simulink model "F28379DFirmware"  (R2023b)
settings: Solver=FixedStepAuto  StartTime=0.0  StopTime=Inf  FixedStep=5e-5  RelTol=1e-3  EnableMultiTasking=on
undefined symbols (not defined in the file): DiscIntNeverNeededParam, Down, F28379D_ADC_MaxCount, F28379D_ADC_Vmax, F28379D_PWM_Counter_Period, Foc_Ki_IxTcpu, Foc_Ki_S, Foc_Kp_I, Foc_Kp_S, GPTRIP1SEL, GPTRIP2SEL, Ia_offset, Ib_offset, IO334_DAC_Vmax, Maxon_645604_Np, PU_System_I_base, PU_System_N_base, Ts_CPU, TZ1, TZ2, Up
libraries: mcbcontrolslib x11, c280xlib x8, canmsglib x7, c2802xlib x6, slpidlib x3, simulink x3, mcbpositiondecoderlib x3, c2837xDlib x3
(part 1 of 2)
settings Model: DataDictionary=PMSM3P2LInverterDd.sldd  EnableAccessToBaseWorkspace=off  ExtModeTrigDuration=8  Creator=mathieu.lu-dac  LastModifiedBy=mathieu.lu-dac
settings OptimizationCC: DefaultUnderspecifiedDataType=single  EnhancedBackFolding=on  PassReuseOutputArgsAs=Individual arguments  MaxStackSize=1024  OptimizeBlockOrder=speed  DifferentSizesBufferReuse=on  OptimizationCustomize=off  DenormalBehavior=FlushToZero  EfficientTunableParamExpr=on
settings DebuggingCC: ParameterTunabilityLossMsg=error
settings HardwareCC: ProdBitPerChar=16  ProdBitPerInt=16  ProdBitPerPointer=32  ProdBitPerSizeT=32  ProdBitPerPtrDiffT=32  ProdLargestAtomicInteger=Integer  ProdLargestAtomicFloat=None  ProdWordSize=16  ProdLongLongMode=on  ProdHWDeviceType=Texas Instruments->C2000
settings SFSimCC: MATLABDynamicMemAlloc=off
settings RTWCC: Description=Embedded Coder  SystemTargetFile=ert.tlc  HardwareBoard=TI Delfino F28379D LaunchPad  TemplateMakefile=ert_default_tmf  Toolchain=Texas Instruments Code Composer Studio (C2000)  PortableWordSizes=on
settings CodeAppCC: ForceParamTrailComments=on  IgnoreCustomStorageClasses=off  OperatorAnnotations=on  SimulinkDataObjDesc=on  SFDataObjDesc=on  InsertBlockDesc=on
settings ERTTargetCC: CodeReplacementLibrary=TI C28x  SupportContinuousTime=on  ExtModeTransport=4  ExtModeStaticAlloc=on  ExtModeAutomaticAllocSize=off  ExtModeMexFile=ext_xcp  ExtModeIntrfLevel=Level2 - Open

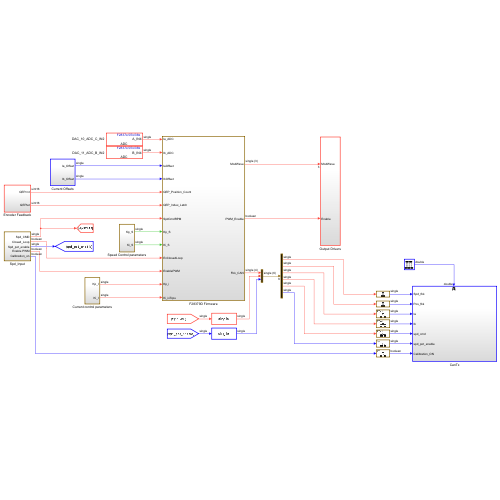
[thumbnail: Simulink's stored preview of the top-level diagram]
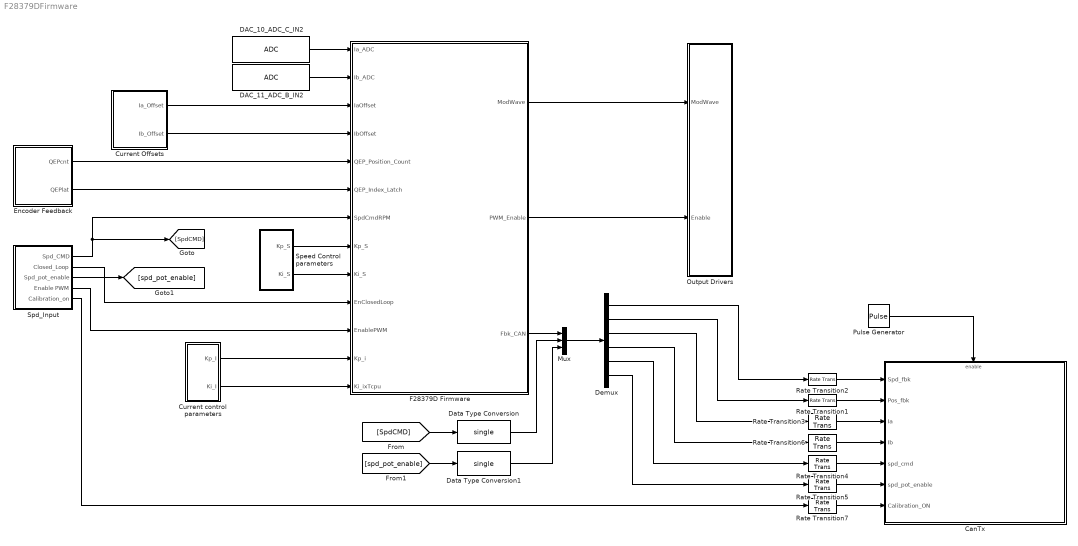
== system F28379DFirmware ==
  CanTx : Subsystem
  Current Offsets : Subsystem
  Current control parameters : Subsystem
  DAC_10_ADC_C_IN2 : c2802xlib/ADC  blkParamProc=C2000_Type4  ADCModule=A  samplingMode=Single sample mode  ADCResolution=12-bit (Single-ended input)  useSOC1=SOC0  useSOC2=SOC0_SOC1  SOCAcquisitionWindow=15  SOCTriggerSource=ePWM1_ADCSOCA  SOCInterruptTrigger=No ADCINT  Ts=-1  dType=single  postInterrupt=off  interruptSel=ADCINT1  ADCINTContinuous=on  endma=off  chdma=1  conv1=ADCINA0  conv2=ADCINA0 and ADCINB0  conv1_Type4=ADCIN4  conv2_Type4=ADCIN0 and ADCIN1
  DAC_11_ADC_B_IN2 : c2802xlib/ADC  blkParamProc=C2000_Type4  ADCModule=B  samplingMode=Single sample mode  ADCResolution=12-bit (Single-ended input)  useSOC1=SOC0  useSOC2=SOC0_SOC1  SOCAcquisitionWindow=15  SOCTriggerSource=ePWM1_ADCSOCA  SOCInterruptTrigger=No ADCINT  Ts=-1  dType=single  postInterrupt=on  interruptSel=ADCINT1  ADCINTContinuous=on  endma=off  chdma=1  conv1=ADCINA0  conv2=ADCINA0 and ADCINB0  conv1_Type4=ADCIN4  conv2_Type4=ADCIN0 and ADCIN1
  Data Type Conversion : DataTypeConversion  OutDataTypeStr=single  SaturateOnIntegerOverflow=off  RndMeth=Floor
  Data Type Conversion1 : DataTypeConversion  OutDataTypeStr=single  SaturateOnIntegerOverflow=off  RndMeth=Floor
  Demux : Demux  Outputs=6
  Encoder Feedback : Subsystem
  F28379D Firmware : Subsystem
  Mux : Mux  Inputs=3
  Output Drivers : Subsystem
  Pulse Generator : DiscretePulseGenerator  Period=10  PulseWidth=5  SampleTime=-1
  Rate Transition{1..7} (7 alike) : RateTransition  OutPortSampleTime=1e-3
  Spd_Input : Subsystem
  Speed Control parameters : Subsystem
  wires:
  Pulse Generator/1 -> CanTx/Enable
  Rate Transition2/1 -> CanTx/1(Spd_fbk)
  Rate Transition1/1 -> CanTx/2(Pos_fbk)
  F28379D Firmware/2(PWM_Enable) -> Output Drivers/2(Enable)
  F28379D Firmware/1(ModWave) -> Output Drivers/1(ModWave)
  Rate Transition3/1 -> CanTx/3(Ia)
  DAC_11_ADC_B_IN2/1 -> F28379D Firmware/2(Ib_ADC)
  DAC_10_ADC_C_IN2/1 -> F28379D Firmware/1(Ia_ADC)
  Spd_Input/1(Spd_CMD) -> F28379D Firmware/7(SpdCmdRPM), [SpdCMD]
  Speed Control parameters/1(Kp_S) -> F28379D Firmware/8(Kp_S)
  Speed Control parameters/2(Ki_S) -> F28379D Firmware/9(Ki_S)
  Spd_Input/2(Closed_Loop) -> F28379D Firmware/10(EnClosedLoop)
  Spd_Input/4(Enable PWM) -> F28379D Firmware/11(EnablePWM)
  Rate Transition4/1 -> CanTx/5(spd_cmd)
  Rate Transition5/1 -> CanTx/6(spd_pot_enable)
  Demux/1 -> Rate Transition2/1
  Demux/2 -> Rate Transition1/1
  Rate Transition6/1 -> CanTx/4("Ib ")
  Demux/5 -> Rate Transition4/1
  Demux/6 -> Rate Transition5/1
  Current Offsets/1(Ia_Offset) -> F28379D Firmware/3(IaOffset)
  Current Offsets/2(Ib_Offset) -> F28379D Firmware/4(IbOffset)
  Demux/3 -> Rate Transition3/1
  Demux/4 -> Rate Transition6/1
  Current control parameters/1(Kp_I) -> F28379D Firmware/12(Kp_i)
  Current control parameters/2(Ki_I) -> F28379D Firmware/13(Ki_ixTcpu)
  Encoder Feedback/1(QEPcnt) -> F28379D Firmware/5(QEP_Position_Count)
  Encoder Feedback/2(QEPlat) -> F28379D Firmware/6(QEP_Index_Latch)
  F28379D Firmware/3(Fbk_CAN) -> Mux/1
  Mux/1 -> Demux/1
  Spd_Input/3(Spd_pot_enable) -> [spd_pot_enable]
  [SpdCMD] -> Data Type Conversion/1
  [spd_pot_enable] -> Data Type Conversion1/1
  Data Type Conversion/1 -> Mux/2
  Data Type Conversion1/1 -> Mux/3
  Spd_Input/5(Calibration_on) -> Rate Transition7/1
  Rate Transition7/1 -> CanTx/7(Calibration_ON)

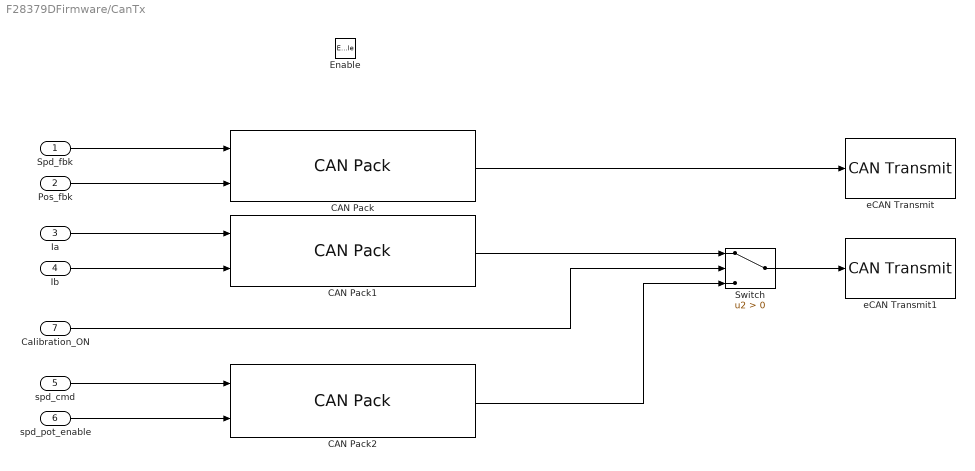
== system F28379DFirmware/CanTx ==
  Spd_fbk : Inport
  Pos_fbk : Inport  Port=2
  Ia : Inport  Port=3
  "Ib " : Inport  Port=4
  spd_cmd : Inport  Port=5
  spd_pot_enable : Inport  Port=6
  Calibration_ON : Inport  Port=7
  Enable : EnablePort
  CAN Pack : canmsglib/CAN Pack  MsgList=(none)  MsgName=Speed_TI_Out  MsgIDType=Standard (11-bit identifier)  MsgIdentifier=1  MsgLength=8  Remote=off  ApplyMinMax=off  BusOutput=off  SignalInfo={ 'Speed_fbk', '0', '32', 'LE', 'single', 'Standard', '0', '1', '0', '-Inf', 'Inf'; 'Pos_fbk', '32', '32', 'LE', 'single', 'Standard', '0', '1', '0', '-Inf', 'Inf' }
      settings: LibrarySourceBlock=canlib/CAN Pack  DataFormat=manually specified signals
  CAN Pack1 : canmsglib/CAN Pack  MsgList=(none)  MsgName=I_TI_Out  MsgIDType=Standard (11-bit identifier)  MsgIdentifier=2  MsgLength=8  Remote=off  ApplyMinMax=off  BusOutput=off  SignalInfo={ 'Ia', '0', '32', 'LE', 'single', 'Standard', '0', '1', '0', '-Inf', 'Inf'; 'Ib', '32', '32', 'LE', 'single', 'Standard', '0', '1', '0', '-Inf', 'Inf' }
      settings: LibrarySourceBlock=canlib/CAN Pack  DataFormat=manually specified signals
  CAN Pack2 : canmsglib/CAN Pack  MsgList=(none)  MsgName=Debug_TI_Out  MsgIDType=Standard (11-bit identifier)  MsgIdentifier=2  MsgLength=8  Remote=off  ApplyMinMax=off  BusOutput=off  SignalInfo={ 'spd_cmd', '0', '32', 'LE', 'single', 'Standard', '0', '1', '0', '-Inf', 'Inf'; 'spd_pot_enable', '32', '32', 'LE', 'single', 'Standard', '0', '1', '0', '-Inf', 'Inf' }
      settings: LibrarySourceBlock=canlib/CAN Pack  DataFormat=manually specified signals
  Switch : Switch  Criteria=u2 > Threshold  SaturateOnIntegerOverflow=off  InputSameDT=off
  eCAN Transmit : c280xlib/CAN Transmit  chipFamily=C280x  useModule=CAN_B  mailboxNo=1  messageID=1  messageType=Standard (11-bit identifier)  enableBlockingMode=off  postInterrupt=off  interruptLine=0
  eCAN Transmit1 : c280xlib/CAN Transmit  chipFamily=C280x  useModule=CAN_B  mailboxNo=1  messageID=2  messageType=Standard (11-bit identifier)  enableBlockingMode=off  postInterrupt=off  interruptLine=0
  wires:
  CAN Pack/1 -> eCAN Transmit/1
  Spd_fbk/1 -> CAN Pack/1
  Pos_fbk/1 -> CAN Pack/2
  Ia/1 -> CAN Pack1/1
  "Ib "/1 -> CAN Pack1/2
  spd_cmd/1 -> CAN Pack2/1
  spd_pot_enable/1 -> CAN Pack2/2
  Switch/1 -> eCAN Transmit1/1
  Calibration_ON/1 -> Switch/2
  CAN Pack1/1 -> Switch/1
  CAN Pack2/1 -> Switch/3

== system F28379DFirmware/Current Offsets ==
  CAN Unpack1 : canmsglib/CAN Unpack  MsgList=(none)  MsgName=CAN Msg  MsgIDType=Standard (11-bit identifier)  MsgIdentifier=30  MsgLength=8  SignalInfo={ 'Ia_off', '0', '32', 'LE', 'single', 'Standard', '0', '1', '0', '-Inf', 'Inf'; 'Ib_off', '32', '32', 'LE', 'single', 'Standard', '0', '1', '0', '-Inf', 'Inf' }  IDPort=off  TimestampPort=off  ErrorPort=off  RemotePort=off  LengthPort=off  StatusPort=off  ApplyMinMax=off
      settings: LibrarySourceBlock=canlib/CAN Unpack
  Data Type Conversion : DataTypeConversion  OutDataTypeStr=single  SaturateOnIntegerOverflow=off  RndMeth=Floor
  Data Type Conversion1 : DataTypeConversion  OutDataTypeStr=single  SaturateOnIntegerOverflow=off  RndMeth=Floor
  Ia Offset : Constant  Value=Ia_offset
  Ib Offset : Constant  Value=Ib_offset
  Switch : Switch  Criteria=u2 ~= 0  SaturateOnIntegerOverflow=off  InputSameDT=off
  Switch1 : Switch  Criteria=u2 ~= 0  SaturateOnIntegerOverflow=off  InputSameDT=off
  eCAN Receive ADC_OFFsets1 : c280xlib/CAN Receive  chipFamily=C280x  useModule=CAN_B  mailboxNo=30  messageID=30  messageType=Standard (11-bit identifier)  enableAcceptanceFiltering=off  messageIDMask=0  sampleTime=0.1  dataType=CAN_MESSAGE_TYPE  outputAction=Output last received values  initValue=0  outputMessageID=off  outputMessageLength=off  outputMessageTimeStamp=off  postInterrupt=off  interruptLine=0
  Ia_Offset : Outport
  Ib_Offset : Outport  Port=2
  wires:
  eCAN Receive ADC_OFFsets1/2 -> CAN Unpack1/1
  Switch/1 -> Data Type Conversion/1
  Switch1/1 -> Data Type Conversion1/1
  Ia Offset/1 -> Switch/3
  Ib Offset/1 -> Switch1/3
  CAN Unpack1/1 -> Switch/2, Switch/1
  CAN Unpack1/2 -> Switch1/1, Switch1/2
  Data Type Conversion/1 -> Ia_Offset/1
  Data Type Conversion1/1 -> Ib_Offset/1

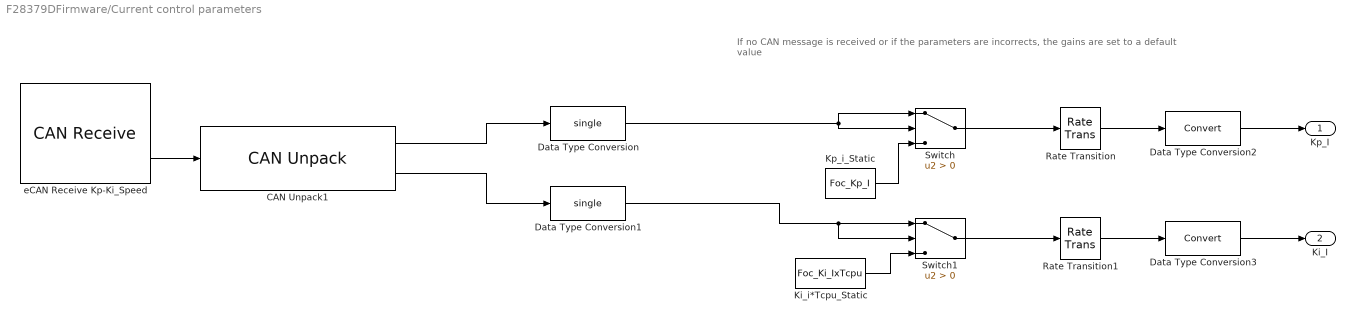
== system F28379DFirmware/Current control parameters ==
  note: If no CAN message is received or if the parameters are incorrects, the gains are set to a default value
  CAN Unpack1 : canmsglib/CAN Unpack  MsgList=(none)  MsgName=CAN Msg  MsgIDType=Standard (11-bit identifier)  MsgIdentifier=29  MsgLength=8  SignalInfo={ 'Kp_I', '0', '32', 'LE', 'single', 'Standard', '0', '1', '0', '-Inf', 'Inf'; 'Ki_I', '32', '32', 'LE', 'single', 'Standard', '0', '1', '0', '-Inf', 'Inf' }  IDPort=off  TimestampPort=off  ErrorPort=off  RemotePort=off  LengthPort=off  StatusPort=off  ApplyMinMax=off
      settings: LibrarySourceBlock=canlib/CAN Unpack
  Data Type Conversion : DataTypeConversion  OutDataTypeStr=single  SaturateOnIntegerOverflow=off  RndMeth=Floor
  Data Type Conversion1 : DataTypeConversion  OutDataTypeStr=single  SaturateOnIntegerOverflow=off  RndMeth=Floor
  Data Type Conversion2 : DataTypeConversion  SaturateOnIntegerOverflow=off  RndMeth=Floor
  Data Type Conversion3 : DataTypeConversion  SaturateOnIntegerOverflow=off  RndMeth=Floor
  Ki_i*Tcpu_Static : Constant  Value=Foc_Ki_IxTcpu  OutDataTypeStr=single  SampleTime=-1
  Kp_i_Static : Constant  Value=Foc_Kp_I  OutDataTypeStr=single  SampleTime=-1
  Rate Transition : RateTransition
  Rate Transition1 : RateTransition  InitialCondition=Ts_CPU
  Switch : Switch  Criteria=u2 > Threshold  SaturateOnIntegerOverflow=off  InputSameDT=off
  Switch1 : Switch  Criteria=u2 > Threshold  SaturateOnIntegerOverflow=off  InputSameDT=off
  eCAN Receive Kp-Ki_Speed : c280xlib/CAN Receive  chipFamily=C280x  useModule=CAN_B  mailboxNo=29  messageID=29  messageType=Standard (11-bit identifier)  enableAcceptanceFiltering=off  messageIDMask=0  sampleTime=1e-3  dataType=CAN_MESSAGE_TYPE  outputAction=Output last received values  initValue=0  outputMessageID=off  outputMessageLength=off  outputMessageTimeStamp=off  postInterrupt=off  interruptLine=0
  Kp_I : Outport
  Ki_I : Outport  Port=2
  wires:
  Data Type Conversion3/1 -> Ki_I/1
  Data Type Conversion2/1 -> Kp_I/1
  Rate Transition1/1 -> Data Type Conversion3/1
  Rate Transition/1 -> Data Type Conversion2/1
  Ki_i*Tcpu_Static/1 -> Switch1/3
  Kp_i_Static/1 -> Switch/3
  Switch1/1 -> Rate Transition1/1
  Switch/1 -> Rate Transition/1
  Data Type Conversion1/1 -> Switch1/1, Switch1/2
  Data Type Conversion/1 -> Switch/2, Switch/1
  CAN Unpack1/2 -> Data Type Conversion1/1
  CAN Unpack1/1 -> Data Type Conversion/1
  eCAN Receive Kp-Ki_Speed/2 -> CAN Unpack1/1

== system F28379DFirmware/Encoder Feedback ==
  Data Type Conversion : DataTypeConversion  OutDataTypeStr=uint16  SaturateOnIntegerOverflow=off  RndMeth=Floor
  Data Type Conversion1 : DataTypeConversion  OutDataTypeStr=uint16  SaturateOnIntegerOverflow=off  RndMeth=Floor
  eQEP : c280xlib/eQEP  useModule=eQEP1  pcInputmode=Quadrature-count  externalClockrate=2x resolution: Count the rising/falling edge  swapPolarityselection=Clockwise  qdfOutputport=off  qapPolarityselection=off  qbpPolarityselection=off  qipPolarityselection=off  qspPolarityselection=off  igatePolarityselection=off  sampleTime=-1  pcOutputport=on  pcMaximumvalue=2^16-1  indexInitializationcheck=off  indexInitializationevent=Rising edge  strobeInitializationcheck=off  strobeInitializationevent=Rising edge  softwareInitializationcheck=off  softwareInitializationsource=Set to init value at start up  softwareInitializationmode=on  pcInitialvalue=2147483648  pcResetmode=Reset on the first index event  ieloutputport=on  indexEventlatch=Falling edge  seloutputport=off  strobeEventlatch=Rising edge  pcefOutputport=off  enableEqepcapture=off  qctmrOutputport=off  qcprdOutputport=off  captureTimerprescaler=128  upEventprescaler=128  overflowErrorflag=off  directionErrorflag=off  captureTimerposition=On position counter read  unitTimerperiod=100000000  captureTimerlatch=off  capturePeriodlatch=off  positionCounterlatch=off  soenPolarityselection=off  spselPolarityselection=Index pin is used for sync output  compareValuesource=Specify via dialog  shadowMode=Load on QPOSCNT=0  compareValue=4294967295  syncOutputwidth=1  polaritySyncoutput=Active high  watchdogEnable=off  watchdogTimer=65535  outport1Datatype=auto  outport2Datatype=auto  outport3Datatype=auto  outport4Datatype=auto  outport5Datatype=auto  outport6Datatype=auto  outport7Datatype=auto  outport8Datatype=auto  outport9Datatype=auto  outport10Datatype=auto  outport11Datatype=auto  outport12Datatype=auto  eqepinterrupt_pce=off  eqepinterrupt_qpe=off  eqepinterrupt_qdc=off  eqepinterrupt_wto=off  eqepinterrupt_pcu=off  eqepinterrupt_pco=off  eqepinterrupt_pcr=off  eqepinterrupt_pcm=off  eqepinterrupt_sel=off  eqepinterrupt_iel=off  eqepinterrupt_uto=off  pheOutputport=off  watchdogOutputport=off  outport13Datatype=auto  outport14Datatype=auto
  QEPcnt : Outport
  QEPlat : Outport  Port=2
  wires:
  eQEP/1 -> Data Type Conversion/1
  eQEP/2 -> Data Type Conversion1/1
  Data Type Conversion1/1 -> QEPlat/1
  Data Type Conversion/1 -> QEPcnt/1

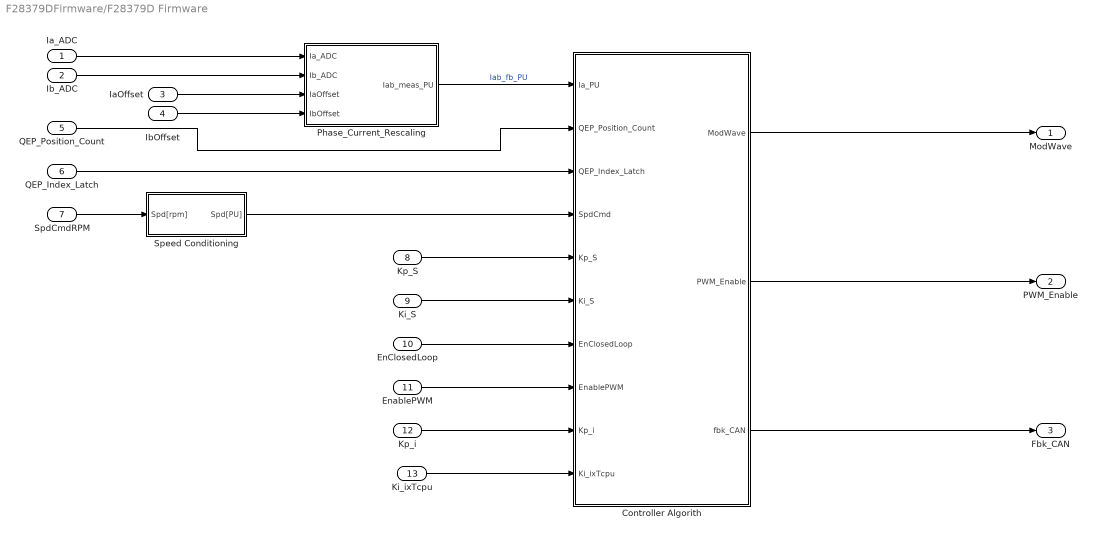
== system F28379DFirmware/F28379D Firmware ==
  Ia_ADC : Inport
  Ib_ADC : Inport  Port=2
  IaOffset : Inport  Port=3
  IbOffset : Inport  Port=4
  QEP_Position_Count : Inport  Port=5
  QEP_Index_Latch : Inport  Port=6
  SpdCmdRPM : Inport  Port=7
  Kp_S : Inport  Port=8
  Ki_S : Inport  Port=9
  EnClosedLoop : Inport  Port=10
  EnablePWM : Inport  Port=11
  Kp_i : Inport  Port=12
  Ki_ixTcpu : Inport  Port=13
  Controller Algorith : Subsystem
  Phase_Current_Rescaling : Subsystem
  Speed Conditioning : Subsystem
  ModWave : Outport
  PWM_Enable : Outport  Port=2
  Fbk_CAN : Outport  Port=3
  wires:
  SpdCmdRPM/1 -> Speed Conditioning/1(Spd[rpm])
  Ia_ADC/1 -> Phase_Current_Rescaling/1(Ia_ADC)
  IaOffset/1 -> Phase_Current_Rescaling/3(IaOffset)
  IbOffset/1 -> Phase_Current_Rescaling/4(IbOffset)
  QEP_Position_Count/1 -> Controller Algorith/2(QEP_Position_Count)
  Controller Algorith/1(ModWave) -> ModWave/1
  Phase_Current_Rescaling/1(Iab_meas_PU) -> Controller Algorith/1(Ia_PU)  "Iab_fb_PU"
  Kp_S/1 -> Controller Algorith/5(Kp_S)
  Controller Algorith/2(PWM_Enable) -> PWM_Enable/1
  Ki_S/1 -> Controller Algorith/6(Ki_S)
  QEP_Index_Latch/1 -> Controller Algorith/3(QEP_Index_Latch)
  Ib_ADC/1 -> Phase_Current_Rescaling/2(Ib_ADC)
  EnClosedLoop/1 -> Controller Algorith/7(EnClosedLoop)
  EnablePWM/1 -> Controller Algorith/8(EnablePWM)
  Speed Conditioning/1(Spd[PU]) -> Controller Algorith/4(SpdCmd)
  Controller Algorith/3(fbk_CAN) -> Fbk_CAN/1
  Kp_i/1 -> Controller Algorith/9(Kp_i)
  Ki_ixTcpu/1 -> Controller Algorith/10(Ki_ixTcpu)

== system F28379DFirmware/Output Drivers ==
  note: for inverter connected with LaunchXL-28379D
  note: System Outputs
  ModWave : Inport
  Enable : Inport  Port=2
  Demux1 : Demux  Outputs=3
  Mux3 : Mux  Inputs=3
  Scale_to_PWM_Counter_PRD : Gain  Gain=F28379D_PWM_Counter_Period  OutDataTypeStr=uint16  RndMeth=Simplest
  Switch1 : Switch  Threshold=0.5  SaturateOnIntegerOverflow=off  InputSameDT=off
  ePWM1 : c2802xlib/ePWM  PwmType=C2000_Type4  useModule=ePWM1  ePWMxLINKTBPRD=Not Linked  periodUnits=Clock cycles  timerSource=Specify via dialog  timerPeriod_clk=F28379D_PWM_Counter_Period+1  timerPeriod_sec=0.0001  tbshadow=Counter equals to zero  countingMode=Up-Down  phaseActiveEnable=Disable  phaseDirection=Count down after sync  phaseActive=0  synchronizationEnable=off  dcaevt1Sync=off  dcbevt1Sync=off  synchronizationOption=Counter equals to zero (CTR=Zero)  dcbevt1SyncOut=off  dcaevt1SyncOut=off  cmpdSyncOut=off  cmpcSyncOut=off  cmpbSyncOut=off  zeroSyncOut=on  swfSyncOut=off  perSynchronizationOption=Counter equals to period (CTR=PRD)  clockPrescale=1  HSclockPrescale=1  enswap=off  ePWMxAStatus=on  ePWMxAactionLogic1=Do nothing  ePWMxAactionLogic2=Do nothing  ePWMxAactionLogic3=Clear  ePWMxAactionLogic4=Set  ePWMxAactionLogic5=Do nothing  ePWMxAactionLogic6=Do nothing  ePWMxACSFenable=off  ePWMxACSFvalue=Forcing disable  ePWMxASFreload=Zero  ePWMxBStatus=on  ePWMxBactionLogic1=Set  ePWMxBactionLogic2=Clear  ePWMxBactionLogic3=Do nothing  ePWMxBactionLogic4=Do nothing  ePWMxBactionLogic5=Clear  ePWMxBactionLogic6=Set  ePWMxBCSFenable=off  ePWMxBCSFvalue=Forcing disable  ePWMxBSFreload=Zero  ePWNxBOutWay=on  ePWMxLINKCMPA=Not Linked  CMPAUnits=Clock cycles  CMPASource=Input port  CMPAValue_per=50  CMPAValue_clk=floor(F28379D_PWM_Counter_Period/2+1)  enCMPAshadow=Counter equals to zero (CTR=Zero)  ePWMxLINKCMPB=Not Linked  CMPBUnits=Clock cycles  CMPBSource=Specify via dialog  CMPBValue_per=50  CMPBValue_clk=floor(F28379D_PWM_Counter_Period/2+1)  enCMPBshadow=Counter equals to zero (CTR=Zero)  ePWMxLINKCMPC=Not Linked  CMPCUnits=Clock cycles  CMPCSource=Specify via dialog  CMPCValue_per=50  CMPCValue_clk=32000  enCMPCshadow=Counter equals to zero (CTR=Zero)  ePWMxLINKCMPD=Not Linked  CMPDUnits=Clock cycles  CMPDSource=Specify via dialog  CMPDValue_per=50  CMPDValue_clk=32000  enCMPDshadow=Counter equals to zero (CTR=Zero)  enableDBePWMxA=on  enableDBePWMxB=on  enhalfcycle=off  DBpolarity=Active high complementary (AHC)  DBedgeDelay=Positive  DBSource_ePWMxA=ePWMxA  DBSource_ePWMxB=ePWMxA  DBPeriodUnits=Clock cycles  DBperiodSource=Specify via dialog  REDperiod=15  FEDperiod=15  REDperiod_sec=0  FEDperiod_sec=0  LoadModeDBRED=Immediate without using shadow  LoadModeDBFED=Immediate without using shadow  adcstartModuleA=on  adcrequestEventA=First event  adcstartEventA=Digital Compare Module A Event 1 start of conversion (DCAEVT1.soc)  adcstartEventA_type2=Counter equals to period (CTR=PRD)  adcstartModuleB=off  adcrequestEventB=First event  adcstartEventB=Counter equals to zero (CTR=Zero)  adcstartEventB_type2=Counter equals to zero (CTR=Zero)  intEn=off  intPrd=First event  intSel=Counter equals to zero (CTR=Zero)  intSel_type2=Counter equals to zero (CTR=Zero)  hrpe=off  enHRPWM=off  HRPWM_LoadMode=Counter equals to period (CTR=PRD)  HRPWM_CTLMode=Duty or Period control mode  HRPWM_EDGMode=Both edge  hrpeb=off  enHRPWMB=off  HRPWM_LoadModeB=Counter equals to zero (CTR=ZERO)  HRPWM_CTLModeB=Duty or Period control mode  HRPWM_EDGModeB=Both edge  enHRDBRED=off  enHRDBFED=off  enSFO=on  enautoconv=on  chopperEnable=off  chopperFrequency=1  chopperFirstwidth=1  chopperDuty=12.5%  tripZonesource=Specify via dialog  tzselOSHT1=off  tzselOSHT2=off  tzselOSHT3=off  tzselOSHDCAEV1=off  tzselOSHDCBEV1=off  tzselCBC1=off  tzselCBC2=off  tzselCBC3=off  tzselCBCDCAEV2=off  tzselCBCDCBEV2=off  tzselOSHT4=off  tzselOSHT5=off  tzselOSHT6=off  tzselCBC4=off  tzselCBC5=off  tzselCBC6=off  enTzOstIntr=off  enTzCbcIntr=off  enTzDCAEVT1Intr=off  enTzDCAEVT2Intr=off  enTzDCBEVT1Intr=off  enTzDCBEVT2Intr=off  ePWMxAforced=No action  ePWMxBforced=No action  DCAEVT1forced=No action  DCBEVT1forced=No action  DCAEVT2forced=No action  DCBEVT2forced=No action  dcah=Trip Zone 1 input (TZ1)  dcal=Trip Zone 2 input (TZ2)  dcbh=Trip Zone 1 input (TZ1)  dcbl=Trip Zone 2 input (TZ2)  dcah_type2=GPTRIP1SEL/(TZ1)  dcal_type2=GPTRIP2SEL/(TZ2)  dcbh_type2=GPTRIP1SEL/(TZ1)  dcbl_type2=GPTRIP2SEL/(TZ2)  gendcaevt1=Event disabled  gendcaevt2=Event disabled  gendcbevt1=Event disabled  gendcbevt2=Event disabled  dcaevt1src=DCAEVT1 with sync  dcaevt2src=DCAEVT2 with sync  dcbevt1src=DCBEVT1 with sync  dcbevt2src=DCBEVT2 with sync  pulsesel=Counter equals to zero (CTR=Zero)  blankinv=off  blankoffset=0  blankwidth=0  evsrcsel=Filtered version of DCAEVT1 (DCAEVT1FILT)  encape=off
  ePWM2 : c2802xlib/ePWM  PwmType=C2000_Type4  useModule=ePWM2  ePWMxLINKTBPRD=Not Linked  periodUnits=Clock cycles  timerSource=Specify via dialog  timerPeriod_clk=F28379D_PWM_Counter_Period+1  timerPeriod_sec=0.0001  tbshadow=Counter equals to zero  countingMode=Up-Down  phaseActiveEnable=Set counter to phase value specified via dialog  phaseDirection=Count up after sync  phaseActive=0  synchronizationEnable=off  dcaevt1Sync=off  dcbevt1Sync=off  synchronizationOption=Pass through (EPWMxSYNCI or SWFSYNC)  dcbevt1SyncOut=off  dcaevt1SyncOut=off  cmpdSyncOut=off  cmpcSyncOut=off  cmpbSyncOut=off  zeroSyncOut=off  swfSyncOut=on  perSynchronizationOption=Counter equals to period (CTR=PRD)  clockPrescale=1  HSclockPrescale=1  enswap=off  ePWMxAStatus=on  ePWMxAactionLogic1=Do nothing  ePWMxAactionLogic2=Do nothing  ePWMxAactionLogic3=Clear  ePWMxAactionLogic4=Set  ePWMxAactionLogic5=Do nothing  ePWMxAactionLogic6=Do nothing  ePWMxACSFenable=off  ePWMxACSFvalue=Forcing disable  ePWMxASFreload=Zero  ePWMxBStatus=on  ePWMxBactionLogic1=Set  ePWMxBactionLogic2=Clear  ePWMxBactionLogic3=Do nothing  ePWMxBactionLogic4=Do nothing  ePWMxBactionLogic5=Clear  ePWMxBactionLogic6=Set  ePWMxBCSFenable=off  ePWMxBCSFvalue=Forcing disable  ePWMxBSFreload=Zero  ePWNxBOutWay=on  ePWMxLINKCMPA=Not Linked  CMPAUnits=Clock cycles  CMPASource=Input port  CMPAValue_per=50  CMPAValue_clk=floor(F28379D_PWM_Counter_Period/2+1)  enCMPAshadow=Counter equals to zero (CTR=Zero)  ePWMxLINKCMPB=Not Linked  CMPBUnits=Clock cycles  CMPBSource=Specify via dialog  CMPBValue_per=50  CMPBValue_clk=floor(F28379D_PWM_Counter_Period/2+1)  enCMPBshadow=Counter equals to zero (CTR=Zero)  ePWMxLINKCMPC=Not Linked  CMPCUnits=Clock cycles  CMPCSource=Specify via dialog  CMPCValue_per=50  CMPCValue_clk=32000  enCMPCshadow=Counter equals to zero (CTR=Zero)  ePWMxLINKCMPD=Not Linked  CMPDUnits=Clock cycles  CMPDSource=Specify via dialog  CMPDValue_per=50  CMPDValue_clk=32000  enCMPDshadow=Counter equals to zero (CTR=Zero)  enableDBePWMxA=on  enableDBePWMxB=on  enhalfcycle=off  DBpolarity=Active high complementary (AHC)  DBedgeDelay=Positive  DBSource_ePWMxA=ePWMxA  DBSource_ePWMxB=ePWMxA  DBPeriodUnits=Clock cycles  DBperiodSource=Specify via dialog  REDperiod=15  FEDperiod=15  REDperiod_sec=0  FEDperiod_sec=0  LoadModeDBRED=Immediate without using shadow  LoadModeDBFED=Immediate without using shadow  adcstartModuleA=off  adcrequestEventA=First event  adcstartEventA=Digital Compare Module A Event 1 start of conversion (DCAEVT1.soc)  adcstartEventA_type2=Counter equals to period (CTR=PRD)  adcstartModuleB=off  adcrequestEventB=First event  adcstartEventB=Counter equals to zero (CTR=Zero)  adcstartEventB_type2=Counter equals to zero (CTR=Zero)  intEn=off  intPrd=First event  intSel=Counter equals to zero (CTR=Zero)  intSel_type2=Counter equals to zero (CTR=Zero)  hrpe=off  enHRPWM=off  HRPWM_LoadMode=Counter equals to period (CTR=PRD)  HRPWM_CTLMode=Duty or Period control mode  HRPWM_EDGMode=Both edge  hrpeb=off  enHRPWMB=off  HRPWM_LoadModeB=Counter equals to zero (CTR=ZERO)  HRPWM_CTLModeB=Duty or Period control mode  HRPWM_EDGModeB=Both edge  enHRDBRED=off  enHRDBFED=off  enSFO=on  enautoconv=on  chopperEnable=off  chopperFrequency=1  chopperFirstwidth=1  chopperDuty=12.5%  tripZonesource=Specify via dialog  tzselOSHT1=off  tzselOSHT2=off  tzselOSHT3=off  tzselOSHDCAEV1=off  tzselOSHDCBEV1=off  tzselCBC1=off  tzselCBC2=off  tzselCBC3=off  tzselCBCDCAEV2=off  tzselCBCDCBEV2=off  tzselOSHT4=off  tzselOSHT5=off  tzselOSHT6=off  tzselCBC4=off  tzselCBC5=off  tzselCBC6=off  enTzOstIntr=off  enTzCbcIntr=off  enTzDCAEVT1Intr=off  enTzDCAEVT2Intr=off  enTzDCBEVT1Intr=off  enTzDCBEVT2Intr=off  ePWMxAforced=No action  ePWMxBforced=No action  DCAEVT1forced=No action  DCBEVT1forced=No action  DCAEVT2forced=No action  DCBEVT2forced=No action  dcah=Trip Zone 1 input (TZ1)  dcal=Trip Zone 2 input (TZ2)  dcbh=Trip Zone 1 input (TZ1)  dcbl=Trip Zone 2 input (TZ2)  dcah_type2=GPTRIP1SEL/(TZ1)  dcal_type2=GPTRIP2SEL/(TZ2)  dcbh_type2=GPTRIP1SEL/(TZ1)  dcbl_type2=GPTRIP2SEL/(TZ2)  gendcaevt1=Event disabled  gendcaevt2=Event disabled  gendcbevt1=Event disabled  gendcbevt2=Event disabled  dcaevt1src=DCAEVT1 with sync  dcaevt2src=DCAEVT2 with sync  dcbevt1src=DCBEVT1 with sync  dcbevt2src=DCBEVT2 with sync  pulsesel=Counter equals to zero (CTR=Zero)  blankinv=off  blankoffset=0  blankwidth=0  evsrcsel=Filtered version of DCAEVT1 (DCAEVT1FILT)  encape=off
  ePWM3 : c2802xlib/ePWM  PwmType=C2000_Type4  useModule=ePWM3  ePWMxLINKTBPRD=Not Linked  periodUnits=Clock cycles  timerSource=Specify via dialog  timerPeriod_clk=F28379D_PWM_Counter_Period+1  timerPeriod_sec=0.0001  tbshadow=Counter equals to zero  countingMode=Up-Down  phaseActiveEnable=Set counter to phase value specified via dialog  phaseDirection=Count up after sync  phaseActive=0  synchronizationEnable=off  dcaevt1Sync=off  dcbevt1Sync=off  synchronizationOption=Pass through (EPWMxSYNCI or SWFSYNC)  dcbevt1SyncOut=off  dcaevt1SyncOut=off  cmpdSyncOut=off  cmpcSyncOut=off  cmpbSyncOut=off  zeroSyncOut=off  swfSyncOut=on  perSynchronizationOption=Counter equals to period (CTR=PRD)  clockPrescale=1  HSclockPrescale=1  enswap=off  ePWMxAStatus=on  ePWMxAactionLogic1=Do nothing  ePWMxAactionLogic2=Do nothing  ePWMxAactionLogic3=Clear  ePWMxAactionLogic4=Set  ePWMxAactionLogic5=Do nothing  ePWMxAactionLogic6=Do nothing  ePWMxACSFenable=off  ePWMxACSFvalue=Forcing disable  ePWMxASFreload=Zero  ePWMxBStatus=on  ePWMxBactionLogic1=Set  ePWMxBactionLogic2=Clear  ePWMxBactionLogic3=Do nothing  ePWMxBactionLogic4=Do nothing  ePWMxBactionLogic5=Clear  ePWMxBactionLogic6=Set  ePWMxBCSFenable=off  ePWMxBCSFvalue=Forcing disable  ePWMxBSFreload=Zero  ePWNxBOutWay=on  ePWMxLINKCMPA=Not Linked  CMPAUnits=Clock cycles  CMPASource=Input port  CMPAValue_per=50  CMPAValue_clk=floor(F28379D_PWM_Counter_Period/2+1)  enCMPAshadow=Counter equals to zero (CTR=Zero)  ePWMxLINKCMPB=Not Linked  CMPBUnits=Clock cycles  CMPBSource=Specify via dialog  CMPBValue_per=50  CMPBValue_clk=floor(F28379D_PWM_Counter_Period+1)  enCMPBshadow=Counter equals to zero (CTR=Zero)  ePWMxLINKCMPC=Not Linked  CMPCUnits=Clock cycles  CMPCSource=Specify via dialog  CMPCValue_per=50  CMPCValue_clk=32000  enCMPCshadow=Counter equals to zero (CTR=Zero)  ePWMxLINKCMPD=Not Linked  CMPDUnits=Clock cycles  CMPDSource=Specify via dialog  CMPDValue_per=50  CMPDValue_clk=32000  enCMPDshadow=Counter equals to zero (CTR=Zero)  enableDBePWMxA=on  enableDBePWMxB=on  enhalfcycle=off  DBpolarity=Active high complementary (AHC)  DBedgeDelay=Positive  DBSource_ePWMxA=ePWMxA  DBSource_ePWMxB=ePWMxA  DBPeriodUnits=Clock cycles  DBperiodSource=Specify via dialog  REDperiod=15  FEDperiod=15  REDperiod_sec=0  FEDperiod_sec=0  LoadModeDBRED=Immediate without using shadow  LoadModeDBFED=Immediate without using shadow  adcstartModuleA=off  adcrequestEventA=First event  adcstartEventA=Digital Compare Module A Event 1 start of conversion (DCAEVT1.soc)  adcstartEventA_type2=Counter equals to period (CTR=PRD)  adcstartModuleB=off  adcrequestEventB=First event  adcstartEventB=Counter equals to zero (CTR=Zero)  adcstartEventB_type2=Counter equals to zero (CTR=Zero)  intEn=off  intPrd=First event  intSel=Counter equals to zero (CTR=Zero)  intSel_type2=Counter equals to zero (CTR=Zero)  hrpe=off  enHRPWM=off  HRPWM_LoadMode=Counter equals to period (CTR=PRD)  HRPWM_CTLMode=Duty or Period control mode  HRPWM_EDGMode=Both edge  hrpeb=off  enHRPWMB=off  HRPWM_LoadModeB=Counter equals to zero (CTR=ZERO)  HRPWM_CTLModeB=Duty or Period control mode  HRPWM_EDGModeB=Both edge  enHRDBRED=off  enHRDBFED=off  enSFO=on  enautoconv=on  chopperEnable=off  chopperFrequency=1  chopperFirstwidth=1  chopperDuty=12.5%  tripZonesource=Specify via dialog  tzselOSHT1=off  tzselOSHT2=off  tzselOSHT3=off  tzselOSHDCAEV1=off  tzselOSHDCBEV1=off  tzselCBC1=off  tzselCBC2=off  tzselCBC3=off  tzselCBCDCAEV2=off  tzselCBCDCBEV2=off  tzselOSHT4=off  tzselOSHT5=off  tzselOSHT6=off  tzselCBC4=off  tzselCBC5=off  tzselCBC6=off  enTzOstIntr=off  enTzCbcIntr=off  enTzDCAEVT1Intr=off  enTzDCAEVT2Intr=off  enTzDCBEVT1Intr=off  enTzDCBEVT2Intr=off  ePWMxAforced=No action  ePWMxBforced=No action  DCAEVT1forced=No action  DCBEVT1forced=No action  DCAEVT2forced=No action  DCBEVT2forced=No action  dcah=Trip Zone 1 input (TZ1)  dcal=Trip Zone 2 input (TZ2)  dcbh=Trip Zone 1 input (TZ1)  dcbl=Trip Zone 2 input (TZ2)  dcah_type2=GPTRIP1SEL/(TZ1)  dcal_type2=GPTRIP2SEL/(TZ2)  dcbh_type2=GPTRIP1SEL/(TZ1)  dcbl_type2=GPTRIP2SEL/(TZ2)  gendcaevt1=Event disabled  gendcaevt2=Event disabled  gendcbevt1=Event disabled  gendcbevt2=Event disabled  dcaevt1src=DCAEVT1 with sync  dcaevt2src=DCAEVT2 with sync  dcbevt1src=DCBEVT1 with sync  dcbevt2src=DCBEVT2 with sync  pulsesel=Counter equals to zero (CTR=Zero)  blankinv=off  blankoffset=0  blankwidth=0  evsrcsel=Filtered version of DCAEVT1 (DCAEVT1FILT)  encape=off
  stop : Constant  Value=0  OutDataTypeStr=uint16
  wires:
  Scale_to_PWM_Counter_PRD/1 -> Switch1/1
  Enable/1 -> Switch1/2  "Active high logic for inverter enable"
  stop/1 -> Mux3/1, Mux3/2, Mux3/3
  Mux3/1 -> Switch1/3
  Switch1/1 -> Demux1/1
  ModWave/1 -> Scale_to_PWM_Counter_PRD/1  "PWM Duty Cycles"
  Demux1/1 -> ePWM1/1  "PWM_A"
  Demux1/2 -> ePWM2/1
  Demux1/3 -> ePWM3/1  "PWM_C"

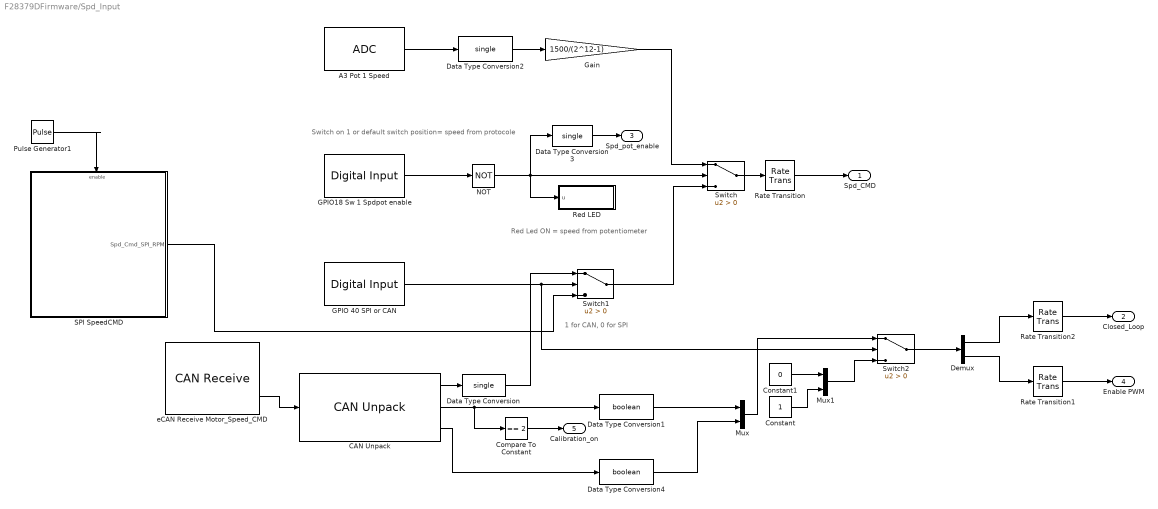
== system F28379DFirmware/Spd_Input ==
  note: Switch on 1 or default switch position= speed from protocole
  note: 1 for CAN, 0 for SPI
  note: Red Led ON = speed from potentiometer
  A3 Pot 1 Speed : c2802xlib/ADC  blkParamProc=C2000_Type4  ADCModule=A  samplingMode=Single sample mode  ADCResolution=12-bit (Single-ended input)  useSOC1=SOC3  useSOC2=SOC0_SOC1  SOCAcquisitionWindow=15  SOCTriggerSource=Software  SOCInterruptTrigger=No ADCINT  Ts=0.1  dType=uint16  postInterrupt=off  interruptSel=ADCINT1  ADCINTContinuous=on  endma=off  chdma=1  conv1=ADCINA0  conv2=ADCINA0 and ADCINB0  conv1_Type4=ADCIN3  conv2_Type4=ADCIN0 and ADCIN1
  CAN Unpack : canmsglib/CAN Unpack  MsgList=(none)  MsgName=CAN Msg  MsgIDType=Standard (11-bit identifier)  MsgIdentifier=0  MsgLength=8  SignalInfo={ 'Speed_Cmd', '0', '32', 'LE', 'single', 'Standard', '0', '1', '0', '-Inf', 'Inf'; 'Closed_Loop', '32', '8', 'LE', 'unsigned', 'Standard', '0', '1', '0', '-Inf', 'Inf'; 'EnablePWM', '40', '8', 'LE', 'unsigned', 'Standard', '0', '1', '0', '-Inf', 'Inf' }  IDPort=off  TimestampPort=off  ErrorPort=off  RemotePort=off  LengthPort=off  StatusPort=off  ApplyMinMax=off
      settings: LibrarySourceBlock=canlib/CAN Unpack
  Compare To Constant : simulink/Logic and Bit Operations/Compare To Constant  relop===  const=2  OutDataTypeStr=boolean
  Constant : Constant  OutDataTypeStr=boolean
  Constant1 : Constant  Value=0  OutDataTypeStr=boolean
  Data Type Conversion : DataTypeConversion  OutDataTypeStr=single  SaturateOnIntegerOverflow=off  RndMeth=Floor
  Data Type Conversion1 : DataTypeConversion  OutDataTypeStr=boolean  SaturateOnIntegerOverflow=off  RndMeth=Floor
  Data Type Conversion2 : DataTypeConversion  OutDataTypeStr=single  SaturateOnIntegerOverflow=off  RndMeth=Floor
  Data Type Conversion3 : DataTypeConversion  OutDataTypeStr=single  SaturateOnIntegerOverflow=off  RndMeth=Floor
  Data Type Conversion4 : DataTypeConversion  OutDataTypeStr=boolean  SaturateOnIntegerOverflow=off  RndMeth=Floor
  Demux : Demux  Outputs=2
  GPIO 40 SPI or CAN : c2837xDlib/Digital Input  GPIO_Number=GPIO40~GPIO47  GPIO_Bit0=on  GPIO_Bit1=off  GPIO_Bit2=off  GPIO_Bit3=off  GPIO_Bit4=off  GPIO_Bit5=off  GPIO_Bit6=off  GPIO_Bit7=off  sampleTime=0.1  dataType=boolean  GPIO_Bit0_Qualification=Sync to SYSCLKOUT  GPIO_Bit1_Qualification=Sync to SYSCLKOUT  GPIO_Bit2_Qualification=Sync to SYSCLKOUT  GPIO_Bit3_Qualification=Sync to SYSCLKOUT  GPIO_Bit4_Qualification=Sync to SYSCLKOUT  GPIO_Bit5_Qualification=Sync to SYSCLKOUT  GPIO_Bit6_Qualification=Sync to SYSCLKOUT  GPIO_Bit7_Qualification=Sync to SYSCLKOUT  Qualification_Period=-1
  GPIO18 Sw 1 Spdpot enable : c2837xDlib/Digital Input  GPIO_Number=GPIO16~GPIO23  GPIO_Bit0=off  GPIO_Bit1=off  GPIO_Bit2=on  GPIO_Bit3=off  GPIO_Bit4=off  GPIO_Bit5=off  GPIO_Bit6=off  GPIO_Bit7=off  sampleTime=0.1  dataType=boolean  GPIO_Bit0_Qualification=Sync to SYSCLKOUT  GPIO_Bit1_Qualification=Sync to SYSCLKOUT  GPIO_Bit2_Qualification=Sync to SYSCLKOUT  GPIO_Bit3_Qualification=Sync to SYSCLKOUT  GPIO_Bit4_Qualification=Sync to SYSCLKOUT  GPIO_Bit5_Qualification=Sync to SYSCLKOUT  GPIO_Bit6_Qualification=Sync to SYSCLKOUT  GPIO_Bit7_Qualification=Sync to SYSCLKOUT  Qualification_Period=-1
  Gain : Gain  Gain=1500/(2^12-1)
  Mux : Mux  Inputs=2
  Mux1 : Mux  Inputs=2
  NOT : Logic  Operator=NOT  IconShape=distinctive  AllPortsSameDT=off  OutDataTypeStr=boolean
  Pulse Generator1 : DiscretePulseGenerator  Period=10  PhaseDelay=5  SampleTime=0.1  VectorParams1D=off
  Rate Transition : RateTransition  OutPortSampleTime=5e-5
  Rate Transition1 : RateTransition
  Rate Transition2 : RateTransition
  Red LED : Subsystem
  SPI SpeedCMD : Subsystem
  Switch : Switch  Criteria=u2 > Threshold  SaturateOnIntegerOverflow=off  InputSameDT=off
  Switch1 : Switch  Criteria=u2 > Threshold  SaturateOnIntegerOverflow=off  InputSameDT=off
  Switch2 : Switch  Criteria=u2 > Threshold  SaturateOnIntegerOverflow=off  InputSameDT=off
  eCAN Receive Motor_Speed_CMD : c280xlib/CAN Receive  chipFamily=C280x  useModule=CAN_B  mailboxNo=0  messageID=0  messageType=Standard (11-bit identifier)  enableAcceptanceFiltering=off  messageIDMask=0  sampleTime=0.1  dataType=CAN_MESSAGE_TYPE  outputAction=Output last received values  initValue=0  outputMessageID=off  outputMessageLength=off  outputMessageTimeStamp=off  postInterrupt=off  interruptLine=0
  Spd_CMD : Outport
  Closed_Loop : Outport  Port=2
  Spd_pot_enable : Outport  Port=3
  Enable PWM : Outport  Port=4
  Calibration_on : Outport  Port=5
  wires:
  Switch/1 -> Rate Transition/1
  eCAN Receive Motor_Speed_CMD/2 -> CAN Unpack/1
  A3 Pot 1 Speed/1 -> Data Type Conversion2/1
  Rate Transition2/1 -> Closed_Loop/1
  Data Type Conversion2/1 -> Gain/1
  CAN Unpack/1 -> Data Type Conversion/1
  GPIO18 Sw 1 Spdpot enable/1 -> NOT/1
  Gain/1 -> Switch/1
  Rate Transition/1 -> Spd_CMD/1
  Data Type Conversion3/1 -> Spd_pot_enable/1
  CAN Unpack/3 -> Data Type Conversion4/1
  Rate Transition1/1 -> Enable PWM/1
  Switch1/1 -> Switch/3
  GPIO 40 SPI or CAN/1 -> Switch1/2, Switch2/2
  Data Type Conversion/1 -> Switch1/1
  CAN Unpack/2 -> Data Type Conversion1/1, Compare To Constant/1
  Compare To Constant/1 -> Calibration_on/1
  Pulse Generator1/1 -> SPI SpeedCMD/Enable
  SPI SpeedCMD/1(Spd_Cmd_SPI_RPM) -> Switch1/3
  Switch2/1 -> Demux/1
  Demux/1 -> Rate Transition2/1
  Demux/2 -> Rate Transition1/1
  Data Type Conversion1/1 -> Mux/1
  Data Type Conversion4/1 -> Mux/2
  Mux/1 -> Switch2/1
  Constant/1 -> Mux1/2
  Constant1/1 -> Mux1/1
  Mux1/1 -> Switch2/3
  NOT/1 -> Switch/2, Data Type Conversion3/1, Red LED/1(u)

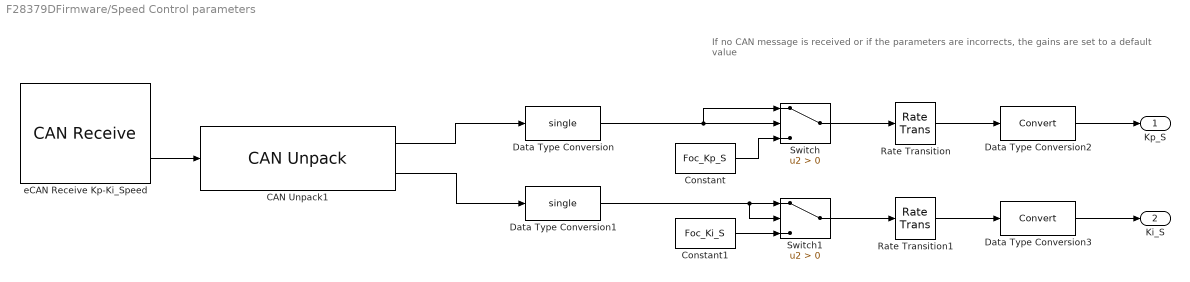
== system F28379DFirmware/Speed Control parameters ==
  note: If no CAN message is received or if the parameters are incorrects, the gains are set to a default value
  CAN Unpack1 : canmsglib/CAN Unpack  MsgList=(none)  MsgName=CAN Msg  MsgIDType=Standard (11-bit identifier)  MsgIdentifier=31  MsgLength=8  SignalInfo={ 'Kp_Speed', '0', '32', 'LE', 'single', 'Standard', '0', '1', '0', '-Inf', 'Inf'; 'Ki_Speed', '32', '32', 'LE', 'single', 'Standard', '0', '1', '0', '-Inf', 'Inf' }  IDPort=off  TimestampPort=off  ErrorPort=off  RemotePort=off  LengthPort=off  StatusPort=off  ApplyMinMax=off
      settings: LibrarySourceBlock=canlib/CAN Unpack
  Constant : Constant  Value=Foc_Kp_S  OutDataTypeStr=single
  Constant1 : Constant  Value=Foc_Ki_S  OutDataTypeStr=single
  Data Type Conversion : DataTypeConversion  OutDataTypeStr=single  SaturateOnIntegerOverflow=off  RndMeth=Floor
  Data Type Conversion1 : DataTypeConversion  OutDataTypeStr=single  SaturateOnIntegerOverflow=off  RndMeth=Floor
  Data Type Conversion2 : DataTypeConversion  SaturateOnIntegerOverflow=off  RndMeth=Floor
  Data Type Conversion3 : DataTypeConversion  SaturateOnIntegerOverflow=off  RndMeth=Floor
  Rate Transition : RateTransition
  Rate Transition1 : RateTransition  InitialCondition=Ts_CPU
  Switch : Switch  Criteria=u2 > Threshold  SaturateOnIntegerOverflow=off  InputSameDT=off
  Switch1 : Switch  Criteria=u2 > Threshold  SaturateOnIntegerOverflow=off  InputSameDT=off
  eCAN Receive Kp-Ki_Speed : c280xlib/CAN Receive  chipFamily=C280x  useModule=CAN_B  mailboxNo=31  messageID=31  messageType=Standard (11-bit identifier)  enableAcceptanceFiltering=off  messageIDMask=0  sampleTime=1e-3  dataType=CAN_MESSAGE_TYPE  outputAction=Output last received values  initValue=0  outputMessageID=off  outputMessageLength=off  outputMessageTimeStamp=off  postInterrupt=off  interruptLine=0
  Kp_S : Outport
  Ki_S : Outport  Port=2
  wires:
  eCAN Receive Kp-Ki_Speed/2 -> CAN Unpack1/1
  CAN Unpack1/1 -> Data Type Conversion/1
  CAN Unpack1/2 -> Data Type Conversion1/1
  Data Type Conversion/1 -> Switch/1, Switch/2
  Data Type Conversion1/1 -> Switch1/2, Switch1/1
  Switch/1 -> Rate Transition/1
  Switch1/1 -> Rate Transition1/1
  Constant/1 -> Switch/3
  Constant1/1 -> Switch1/3
  Rate Transition/1 -> Data Type Conversion2/1
  Rate Transition1/1 -> Data Type Conversion3/1
  Data Type Conversion2/1 -> Kp_S/1
  Data Type Conversion3/1 -> Ki_S/1

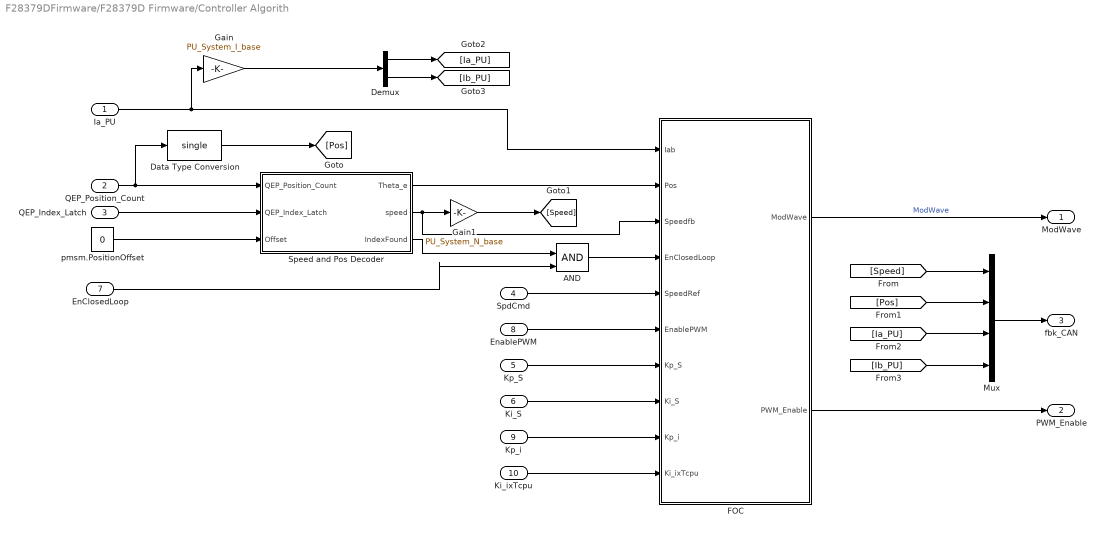
== system F28379DFirmware/F28379D Firmware/Controller Algorith ==
  Ia_PU : Inport
  QEP_Position_Count : Inport  Port=2
  QEP_Index_Latch : Inport  Port=3
  SpdCmd : Inport  Port=4
  Kp_S : Inport  Port=5
  Ki_S : Inport  Port=6
  EnClosedLoop : Inport  Port=7
  EnablePWM : Inport  Port=8
  Kp_i : Inport  Port=9
  Ki_ixTcpu : Inport  Port=10
  AND : Logic  IconShape=distinctive  AllPortsSameDT=off  OutDataTypeStr=boolean
  Data Type Conversion : DataTypeConversion  OutDataTypeStr=single  SaturateOnIntegerOverflow=off  RndMeth=Floor
  Demux : Demux  Outputs=2
  FOC : Subsystem
  Gain : Gain  Gain=PU_System_I_base
  Gain1 : Gain  Gain=PU_System_N_base
  Mux : Mux
  Speed and Pos Decoder : Subsystem
  pmsm.PositionOffset : Constant  Value=0  SampleTime=-1
  ModWave : Outport
  PWM_Enable : Outport  Port=2
  fbk_CAN : Outport  Port=3
  wires:
  EnClosedLoop/1 -> AND/2
  Speed and Pos Decoder/1(Theta_e) -> FOC/2(Pos)
  Ia_PU/1 -> FOC/1(Iab), Gain/1
  EnablePWM/1 -> FOC/6(EnablePWM)
  Speed and Pos Decoder/3(IndexFound) -> AND/1
  AND/1 -> FOC/4(EnClosedLoop)
  pmsm.PositionOffset/1 -> Speed and Pos Decoder/3(Offset)
  Speed and Pos Decoder/2(speed) -> FOC/3(Speedfb), Gain1/1
  FOC/2(PWM_Enable) -> PWM_Enable/1
  QEP_Index_Latch/1 -> Speed and Pos Decoder/2(QEP_Index_Latch)
  FOC/1(ModWave) -> ModWave/1  "ModWave"
  Kp_S/1 -> FOC/7(Kp_S)
  Ki_S/1 -> FOC/8(Ki_S)
  SpdCmd/1 -> FOC/5(SpeedRef)
  [Speed] -> Mux/1
  [Pos] -> Mux/2
  Mux/1 -> fbk_CAN/1
  [Ia_PU] -> Mux/3
  [Ib_PU] -> Mux/4
  Demux/1 -> [Ia_PU]
  Demux/2 -> [Ib_PU]
  Kp_i/1 -> FOC/9(Kp_i)
  Ki_ixTcpu/1 -> FOC/10(Ki_ixTcpu)
  Gain/1 -> Demux/1
  Gain1/1 -> [Speed]
  QEP_Position_Count/1 -> Data Type Conversion/1, Speed and Pos Decoder/1(QEP_Position_Count)
  Data Type Conversion/1 -> [Pos]

== system F28379DFirmware/F28379D Firmware/Phase_Current_Rescaling ==
  Ia_ADC : Inport
  Ib_ADC : Inport  Port=2
  IaOffset : Inport  Port=3
  IbOffset : Inport  Port=4
  ADCtoA : Gain  Gain=10/IO334_DAC_Vmax/IO334_iDAC_gain  RndMeth=Simplest  OutDataTypeStr=Inherit: Same as input
  Add : Sum  Inputs=+-
  Add Constant : Bias  Bias=-2^11*IO334_DAC_Vmax/F28379D_ADC_Vmax  SaturateOnIntegerOverflow=off
  Get ADC Voltage : Gain  Gain=F28379D_ADC_Vmax/F28379D_ADC_MaxCount  OutDataTypeStr=single  RndMeth=Simplest
  Mux : Mux  Inputs=2
  Mux1 : Mux  Inputs=2
  PU_Conversion : Gain  Gain=1/PU_System_I_base  RndMeth=Simplest  OutDataTypeStr=Inherit: Same as input
  Rate Transition : RateTransition
  Iab_meas_PU : Outport  VectorParamsAs1DForOutWhenUnconnected=off
  wires:
  Mux1/1 -> Rate Transition/1
  Ia_ADC/1 -> Mux/1
  Ib_ADC/1 -> Mux/2
  Mux/1 -> Add Constant/1
  PU_Conversion/1 -> Iab_meas_PU/1
  IaOffset/1 -> Mux1/1
  IbOffset/1 -> Mux1/2
  Add Constant/1 -> Get ADC Voltage/1
  Get ADC Voltage/1 -> ADCtoA/1  "Currents_inDACvoltages"
  Rate Transition/1 -> Add/2
  ADCtoA/1 -> Add/1  "Currents_A"
  Add/1 -> PU_Conversion/1  "Currents_no_offset"

== system F28379DFirmware/F28379D Firmware/Speed Conditioning ==
  Spd[rpm] : Inport
  hz2pu : Gain  Gain=60/(PU_System_N_base *Maxon_645604_Np)  RndMeth=Simplest  OutDataTypeStr=Inherit: Same as input
  rads2hz : Gain  Gain=Maxon_645604_Np/(2*pi)
  rmp2rads : Gain  Gain=2*pi/60
  Spd[PU] : Outport
  wires:
  Spd[rpm]/1 -> rmp2rads/1
  rmp2rads/1 -> rads2hz/1
  rads2hz/1 -> hz2pu/1
  hz2pu/1 -> Spd[PU]/1

== system F28379DFirmware/Spd_Input/Red LED ==
  u : Inport
  NOT : Logic  Operator=NOT  IconShape=distinctive  AllPortsSameDT=off  OutDataTypeStr=boolean
  Red LED : c2837xDlib/Digital Output  GPIO_Number=GPIO32~GPIO39  GPIO_Bit0=off  GPIO_BIT0_Toggle=off  GPIO_Bit1=off  GPIO_BIT1_Toggle=off  GPIO_Bit2=on  GPIO_BIT2_Toggle=off  GPIO_Bit3=off  GPIO_BIT3_Toggle=off  GPIO_Bit4=off  GPIO_BIT4_Toggle=off  GPIO_Bit5=off  GPIO_BIT5_Toggle=off  GPIO_Bit6=off  GPIO_BIT6_Toggle=off  GPIO_Bit7=off  GPIO_BIT7_Toggle=off
  wires:
  u/1 -> NOT/1
  NOT/1 -> Red LED/1

== system F28379DFirmware/Spd_Input/SPI SpeedCMD ==
  Enable : EnablePort
  SPI Receive : c280xlib/SPI Receive  SPISelect=SPI_A  ClockPolarity=Rising_edge  ClockPhase=Delay_half_cycle  SPIModule=uint32(0)  Mode=Master  BusSpeed=uint32(1000000)  FirstBitToTransfer=Most significant bit (MSB)  ClockMode=0  BlockFunction=Read  EnableRegisterAddress=on  RegisterAddress=0  OutputDataType=uint16  OutputDataLength=1  BlockingMode=off  SampleTime=0.1  DataBits=16  UseCustomSSPin=Provided by the SPI peripheral  ActiveLowSSPin=Active low  Pin=0
      settings: LibrarySourceBlock=c2837xDlib/SPI Receive
  Uint16toSingle Max Speed 10000 rpm : Subsystem
  Spd_Cmd_SPI_RPM : Outport
  wires:
  SPI Receive/1 -> Uint16toSingle Max Speed 10000 rpm/1(SpeedUnint16)
  Uint16toSingle Max Speed 10000 rpm/1(Spd_Single) -> Spd_Cmd_SPI_RPM/1

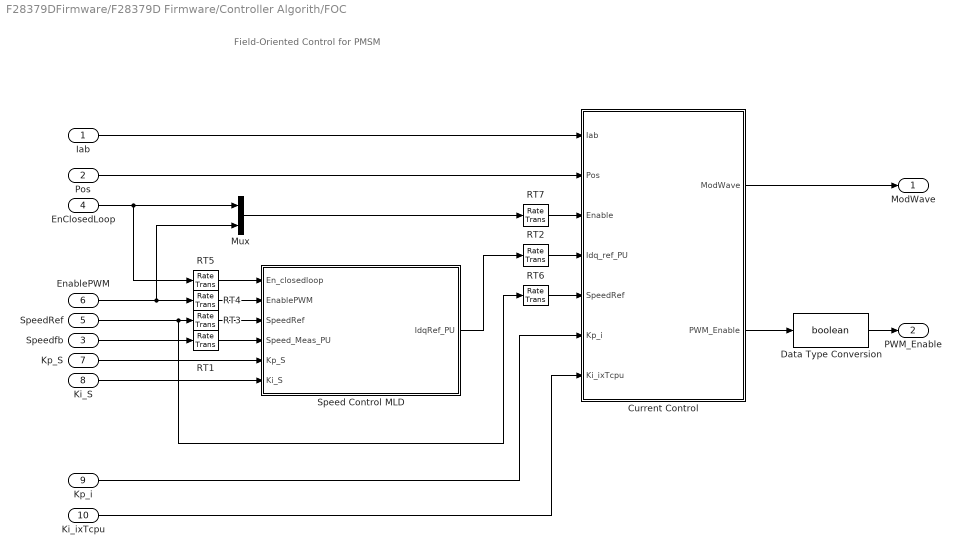
== system F28379DFirmware/F28379D Firmware/Controller Algorith/FOC ==
  note: Field-Oriented Control for PMSM
  Iab : Inport
  Pos : Inport  Port=2
  Speedfb : Inport  Port=3
  EnClosedLoop : Inport  Port=4
  SpeedRef : Inport  Port=5
  EnablePWM : Inport  Port=6
  Kp_S : Inport  Port=7
  Ki_S : Inport  Port=8
  Kp_i : Inport  Port=9
  Ki_ixTcpu : Inport  Port=10
  Current Control : Subsystem  TreatAsAtomicUnit=on
  Data Type Conversion : DataTypeConversion  OutDataTypeStr=boolean  SaturateOnIntegerOverflow=off  RndMeth=Floor
  Mux : Mux  Inputs=2
  RT{1,3..5} (4 alike) : RateTransition  Deterministic=off  OutPortSampleTime=Ts_speed
  RT2 : RateTransition  Deterministic=off
  RT6 : RateTransition  Deterministic=off
  RT7 : RateTransition  Deterministic=off
  Speed Control MLD : Subsystem
  ModWave : Outport
  PWM_Enable : Outport  Port=2
  wires:
  Speed Control MLD/1(IdqRef_PU) -> RT2/1
  EnClosedLoop/1 -> Mux/1, RT5/1
  Speedfb/1 -> RT1/1
  Current Control/2(PWM_Enable) -> Data Type Conversion/1
  EnablePWM/1 -> Mux/2, RT4/1
  Ki_S/1 -> Speed Control MLD/6(Ki_S)
  Current Control/1(ModWave) -> ModWave/1
  Iab/1 -> Current Control/1(Iab)
  Kp_S/1 -> Speed Control MLD/5(Kp_S)
  Pos/1 -> Current Control/2(Pos)
  SpeedRef/1 -> RT6/1, RT3/1
  Mux/1 -> RT7/1
  RT2/1 -> Current Control/4(Idq_ref_PU)
  RT6/1 -> Current Control/5(SpeedRef)
  RT7/1 -> Current Control/3(Enable)
  RT1/1 -> Speed Control MLD/4(Speed_Meas_PU)
  RT3/1 -> Speed Control MLD/3(SpeedRef)
  Data Type Conversion/1 -> PWM_Enable/1
  RT5/1 -> Speed Control MLD/1(En_closedloop)
  RT4/1 -> Speed Control MLD/2(EnablePWM)
  Kp_i/1 -> Current Control/6(Kp_i)
  Ki_ixTcpu/1 -> Current Control/7(Ki_ixTcpu)

== system F28379DFirmware/F28379D Firmware/Controller Algorith/Speed and Pos Decoder ==
  QEP_Position_Count : Inport
  QEP_Index_Latch : Inport  Port=2
  Offset : Inport  Port=3
  Delay : Delay  DelayLength=1
  IIR Filter : mcbcontrolslib/IIR Filter  VariantControl=Low Pass Filter  VariantSelect=Low-pass  Filter_constant=0.01  advancedSettings=off  Ts=50e-6  cutOff_freq=32.1525
  IndexFinder : Subsystem
  Mechanical to Electrical Position : mcbpositiondecoderlib/Mechanical to Electrical Position  PolePairsInputType=Specify via dialog  NrPP=Maxon_645604_Np  selectedRange=Per unit  MechOfstInputType=Input port  mechOffsetIn=0  maxAngleIn=1  InputDataType=single  VariantSelect=floating-point
  NOT : Logic  Operator=NOT  AllPortsSameDT=off  OutDataTypeStr=boolean
  Quadrature Decoder : mcbpositiondecoderlib/Quadrature Decoder  EncoderSlitsPerRevolution=Maxon_Mile_Nslits  EncoderCountsPerSlit=4  CounterSize=16 bits  ExternalIndexCount=on  PositionUnit=Per unit  PositionDataType=single  ParameterInputType=off  CountsPerRevInverseDataType=single
  Speed Measurement : mcbpositiondecoderlib/Speed Measurement  PositionUnit=Per unit  PositionScalingDatatype=uint32  SpeedCalculationMode=Time interval for speed calculation  SampleTimeAsync=Ts_CPU  MaximumApplicationSpeed=6000  SpeedResolution=5e-6  DelayLength=20  MaximumMeasurableSpeed=29999  MeasurableSpeedResolution=1.397e-05  SpeedUnit=Per unit based on dialog  PerUnitSpeed=PU_System_N_base  SpeedDataType=single
  Theta_e : Outport  VectorParamsAs1DForOutWhenUnconnected=off
  speed : Outport  Port=2  VectorParamsAs1DForOutWhenUnconnected=off
  IndexFound : Outport  Port=3  VectorParamsAs1DForOutWhenUnconnected=off
  wires:
  Mechanical to Electrical Position/1 -> Theta_e/1  "Pos"
  Speed Measurement/1 -> IIR Filter/1
  Quadrature Decoder/1 -> Speed Measurement/1, Mechanical to Electrical Position/1
  QEP_Position_Count/1 -> Quadrature Decoder/1
  Offset/1 -> Mechanical to Electrical Position/2
  IIR Filter/1 -> speed/1
  NOT/1 -> IndexFinder/Enable
  QEP_Index_Latch/1 -> IndexFinder/1(In1), Quadrature Decoder/2
  Delay/1 -> NOT/1
  IndexFinder/1(IndexFound) -> IndexFound/1, Delay/1

== system F28379DFirmware/Spd_Input/SPI SpeedCMD/Uint16toSingle Max Speed 10000 rpm ==
  note: Max Speed = 10000 rpm
      | Min Speed = -10000 rpm
  SpeedUnint16 : Inport
  Add Constant : Bias  Bias=-10000  SaturateOnIntegerOverflow=off
  Data Type Conversion2 : DataTypeConversion  OutDataTypeStr=single  SaturateOnIntegerOverflow=off  RndMeth=Floor
  Gain : Gain  Gain=10000/2^15
  Spd_Single : Outport
  wires:
  Gain/1 -> Add Constant/1
  Add Constant/1 -> Spd_Single/1
  SpeedUnint16/1 -> Data Type Conversion2/1
  Data Type Conversion2/1 -> Gain/1

== system F28379DFirmware/F28379D Firmware/Controller Algorith/FOC/Current Control ==
  Iab : Inport
  Pos : Inport  Port=2
  Enable : Inport  Port=3
  Idq_ref_PU : Inport  Port=4
  SpeedRef : Inport  Port=5
  Kp_i : Inport  Port=6
  Ki_ixTcpu : Inport  Port=7
  Control_System : Subsystem
  Terminator : Terminator
  ModWave : Outport  VectorParamsAs1DForOutWhenUnconnected=off
  PWM_Enable : Outport  Port=2  VectorParamsAs1DForOutWhenUnconnected=off
  wires:
  Idq_ref_PU/1 -> Control_System/4(Idq_ref_PU)  "Idq_ref"
  Pos/1 -> Control_System/2(Pos_PU)  "Pos_PU"
  Enable/1 -> Control_System/3(Enable)
  Iab/1 -> Control_System/1(Iab_meas_PU)  "Iab"
  SpeedRef/1 -> Control_System/5(SpeedRef)
  Control_System/1(ModWave) -> ModWave/1
  Control_System/2(PWM_Enable) -> PWM_Enable/1
  Kp_i/1 -> Control_System/6(Kp_i)
  Ki_ixTcpu/1 -> Control_System/7(Ki_ixTcpu)
  Control_System/3(Idq_debug) -> Terminator/1

== system F28379DFirmware/F28379D Firmware/Controller Algorith/FOC/Speed Control MLD ==
  En_closedloop : Inport
  EnablePWM : Inport  Port=2
  SpeedRef : Inport  Port=3
  Speed_Meas_PU : Inport  Port=4
  Kp_S : Inport  Port=5
  Ki_S : Inport  Port=6
  AND : Logic  IconShape=distinctive  AllPortsSameDT=off  OutDataTypeStr=boolean
  Id_Ref : Constant  Value=0  OutDataTypeStr=single
  Mux : Mux  Inputs=2
  PI_Controller_Speed : Subsystem
  Speed_Ref_Selector : Subsystem
  IdqRef_PU : Outport  VectorParamsAs1DForOutWhenUnconnected=off
  wires:
  Mux/1 -> IdqRef_PU/1
  En_closedloop/1 -> AND/1, PI_Controller_Speed/1(Enable)
  Kp_S/1 -> PI_Controller_Speed/4(Kp_S)
  EnablePWM/1 -> AND/2
  Speed_Ref_Selector/1(Speed_Ref_PU) -> PI_Controller_Speed/2(N_ref)
  PI_Controller_Speed/1(Iq_ref) -> Mux/2
  SpeedRef/1 -> Speed_Ref_Selector/2(SpeedCommand)
  AND/1 -> Speed_Ref_Selector/1(Enable)
  Speed_Meas_PU/1 -> PI_Controller_Speed/3(N_fb), Speed_Ref_Selector/3(Speed_Ref_Open)
  Id_Ref/1 -> Mux/1
  Ki_S/1 -> PI_Controller_Speed/5(Ki_S)
